simulink model "PID3"  (R2020b)
settings: Solver=VariableStepAuto  StartTime=0.0  StopTime=120  RelTol=1e-3
undefined symbols (not defined in the file or in its folder): Kd, Ki, Kp
settings Model: DataDictionary=Data.sldd  Creator=vigne  LastModifiedBy=vigne
settings DataIOCC: SaveOutput=off  SaveTime=off

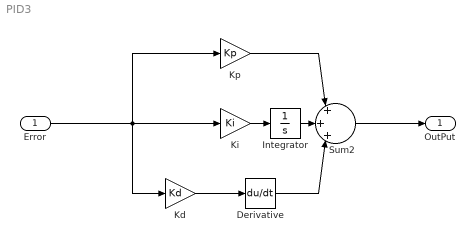
== system PID3 ==
  Error : Inport  OutDataTypeStr=double  PortDimensions=1  SampleTime=0
  Derivative : Derivative
  Integrator : Integrator
  Kd : Gain  Gain=Kd
  Ki : Gain  Gain=Ki
  Kp : Gain  Gain=Kp
  Sum2 : Sum  Inputs=|+|+|+|
  OutPut : Outport  OutDataTypeStr=double  PortDimensions=1  SampleTime=0
  wires:
  Derivative/1 -> Sum2/3
  Kp/1 -> Sum2/1
  Error/1 -> Ki/1, Kp/1, Kd/1
  Kd/1 -> Derivative/1
  Integrator/1 -> Sum2/2
  Ki/1 -> Integrator/1
  Sum2/1 -> OutPut/1
